simulink library "cdmaprivate"  (Simulink 4.00)
libraries: dspsrcs3 x3, dspsigattribs x2, dspmlti3 x2, dspmtrx3 x1
settings Model: CovMetricSettings=d  Creator=akansal  LastModifiedBy=akansal

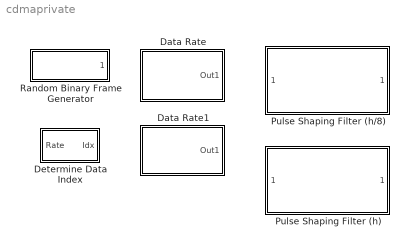
== system cdmaprivate ==
  Data Rate : Subsystem  mask(Base Station Transmitter Data Rate){rate=Full}
      mask prompts: rate "Data Rate"
      mask help: Select the Base Station Transmitter Data Rate.
      settings: RTWFcnNameOpts=Auto  RTWFileNameOpts=Auto
      mask StyleString: popup(Full|Half|Quarter|One-Eighth)
      mask Display: disp('Base Station \nTransmitter\nData Rate')
  Data Rate1 : Subsystem  mask(Mobile Station Transmitter Data Rate){rate=Full}
      mask prompts: rate "Data Rate"
      mask help: Select the Mobile Station Transmitter Data Rate.
      settings: RTWFcnNameOpts=Auto  RTWFileNameOpts=Auto
      mask StyleString: popup(Full|Half|Quarter|One-Eighth)
      mask Display: disp('Mobile Station \nTransmitter \nData Rate')
  Determine Data Index : Subsystem  mask(Determine Data Index){rateSet=Rate Set I}
      mask prompts: rateSet "Rate set:"
      mask help: Deterime index of valid data in the frame based upon rate set and rate input.
      mask init:
      | if(rateSet==1)
      | % --- Rate Set 1
      |    R1F = buffer(1:172,268);
      |    R1H = buffer(1:80,268);
      |    R1Q = buffer(1:40,268);
      |    R1E = buffer(1:16,268);
      |    idxMat = [R1F R1H R1Q R1E];
      | else
      |    % --- Rate Set 2
      |    R2F = [1:268]';
      |    R2H = buffer(1:126,268);
      |    R2Q = buffer(1:56,268);
      |    R2E = buffer(1:22,268);
      |    idxMat = [R2F R2H R2Q R2E];
      | end;
      settings: RTWFcnNameOpts=Auto  RTWFileNameOpts=Auto
      mask StyleString: popup(Rate Set I|Rate Set II)
  Pulse Shaping Filter (h) : Subsystem  mask(FIR Pulse Shaping Filter){N=8}
      mask prompts: N "Interpolation factor:"
      mask help: The length of the FIR filter is the duration of 12 PN sequence chips. The coefficient spacing and the sample time of this filter is one-eighth of the PN sequence chip duration, resulting in a total of 96 coefficients. The filter introduces a delay of 48 samples.
      mask init:
      | load txfiltx8.mat;
      | h = (TxFiltCoefx8*N);
      settings: RTWFcnNameOpts=Auto  RTWFileNameOpts=Auto
      mask Display: plot( 1:prod( size( h)), h);
  Pulse Shaping Filter (h/8) : Subsystem  mask(FIR Pulse Shaping Filter){N=8}
      mask prompts: N "Interpolation factor:"
      mask help: The length of the FIR filter is the duration of 12 PN sequence chips. The coefficient spacing and the sample time of this filter is one-eighth of the PN sequence chip duration, resulting in a total of 96 coefficients. The filter introduces a delay of 48 samples.
      mask init:
      | load txfiltx8.mat;
      | h = (TxFiltCoefx8*N)/8;
      settings: RTWFcnNameOpts=Auto  RTWFileNameOpts=Auto
      mask Display: plot( 1:prod( size( h)), h);
  Random Binary Frame Generator : Subsystem  mask(Random Binary Frame Generator){seed=119940, Ts=1/(50*268), N=268}
      mask prompts: seed "Initial seed:"; Ts "Sample time (sec):"; N "Output frame size:"
      mask help:
      | Generate a random frame of binary integers. The output frame period is
      | (Sample time) * (Output frame size).
      settings: RTWFcnNameOpts=Auto  RTWFileNameOpts=Auto
      mask Display: plot(0,0,100,100,[95,90,90,80,80,60,60,30,30,20,20,10,10,5],[25,25,75,75,25,25,75,75,25,25,75,75,25,25]);

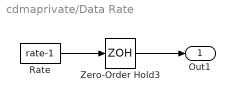
== system cdmaprivate/Data Rate ==
  Rate : Constant  Value=rate-1
  Zero-Order Hold3 : ZeroOrderHold  SampleTime=1/50
  Out1 : Outport  Port=1  InitialOutput=0
  wires:
  Zero-Order Hold3/1 -> Out1/1
  Rate/1 -> Zero-Order Hold3/1

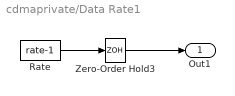
== system cdmaprivate/Data Rate1 ==
  Rate : Constant  Value=rate-1
  Zero-Order Hold3 : ZeroOrderHold  SampleTime=1/50
  Out1 : Outport  Port=1  InitialOutput=0
  wires:
  Zero-Order Hold3/1 -> Out1/1
  Rate/1 -> Zero-Order Hold3/1

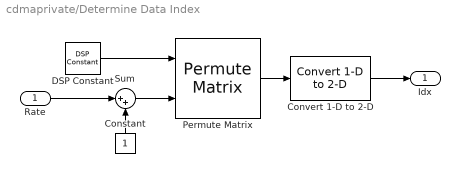
== system cdmaprivate/Determine Data Index ==
  Rate : Inport  Port=1
  Constant : Constant  Orientation=up  Value=1
  Convert 1-D to 2-D : dspsigattribs/Convert 1-D to 2-D  M=268  N=1  frameBasedOut=off
  DSP Constant : dspsrcs3/DSP Constant  Value=idxMat  InterpretAs1D=on  SampleMode=Discrete  Ts=-1  FramebasedOutput=off
  Permute Matrix : dspmtrx3/Permute Matrix  mode=Columns  errmode=Clip Index  checkDims=off
  Sum : Sum  Inputs=|++  SaturateOnIntegerOverflow=on
  Idx : Outport  Port=1
  wires:
  Constant/1 -> Sum/2
  DSP Constant/1 -> Permute Matrix/1
  Permute Matrix/1 -> Convert 1-D to 2-D/1
  Sum/1 -> Permute Matrix/2
  Rate/1 -> Sum/1
  Convert 1-D to 2-D/1 -> Idx/1

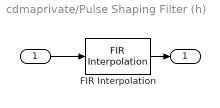
== system cdmaprivate/Pulse Shaping Filter (h) ==
  "   " : Inport  Port=1
  FIR Interpolation : dspmlti3/FIR Interpolation  h=h  L=N  framing=Maintain input frame rate
  " " : Outport  Port=1
  wires:
  "   "/1 -> FIR Interpolation/1
  FIR Interpolation/1 -> " "/1

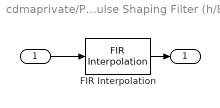
== system cdmaprivate/Pulse Shaping Filter (h/8) ==
  "   " : Inport  Port=1
  FIR Interpolation : dspmlti3/FIR Interpolation  h=h  L=N  framing=Maintain input frame rate
  " " : Outport  Port=1
  wires:
  FIR Interpolation/1 -> " "/1
  "   "/1 -> FIR Interpolation/1

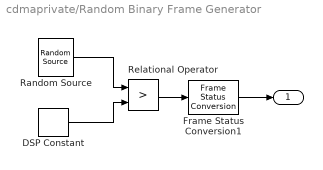
== system cdmaprivate/Random Binary Frame Generator ==
  DSP Constant : dspsrcs3/DSP Constant  Value=0.5  InterpretAs1D=on  SampleMode=Discrete  Ts=Ts*N  FramebasedOutput=off
  Frame Status Conversion1 : dspsigattribs/Frame Status Conversion  growRefPort=off  outframe=Frame-based
  Random Source : dspsrcs3/Random Source  SrcType=Uniform  Min=0  Max=1  Mean=0  Var=1  Seed=seed  Inherit=off  SampMode=Discrete  SampTime=Ts  SampFrame=N  OutComplex=Real
  Relational Operator : RelationalOperator  Operator=>
  " " : Outport  Port=1
  wires:
  Frame Status Conversion1/1 -> " "/1
  Relational Operator/1 -> Frame Status Conversion1/1
  DSP Constant/1 -> Relational Operator/2
  Random Source/1 -> Relational Operator/1
